simulink model "CubeRF"  (R2020b)
settings: Solver=FixedStepAuto  StartTime=0.0  StopTime=inf  FixedStep=0.05  RelTol=1e-3
undefined symbols (not defined in the file): Pose, Twist
libraries: robotlib x3
settings Model: Creator=iris  LastModifiedBy=iris
settings OptimizationCC: EnhancedBackFolding=on  PassReuseOutputArgsAs=Individual arguments  ZeroExternalMemoryAtStartup=off  ZeroInternalMemoryAtStartup=off  MaxStackSize=64  OptimizeBlockOrder=speed  DifferentSizesBufferReuse=on  OptimizationCustomize=off  EfficientTunableParamExpr=on
settings DebuggingCC: ParameterTunabilityLossMsg=error  SFMachineParentedDataDiag=error
settings HardwareCC: ProdBitPerPointer=32  ProdBitPerSizeT=32  ProdBitPerPtrDiffT=32  ProdLargestAtomicFloat=None  ProdIntDivRoundTo=Undefined  ProdEndianess=Unspecified  ProdWordSize=32  ProdHWDeviceType=Generic->Unspecified (assume 32-bit Generic)
settings SFSimCC: MATLABDynamicMemAlloc=off  SimTargetLang=C++
settings RTWCC: Description=Embedded Coder  SystemTargetFile=ert.tlc  HardwareBoard=Robot Operating System (ROS)  TLCOptions="-aInlineSetEventsForThisBaseRateFcn=TLC_FALSE -aSuppressMultiTaskScheduler=TLC_FALSE  -aRateBasedStepFcn=0"  TemplateMakefile=ert_default_tmf  Toolchain=Catkin  TargetLang=C++
settings CodeAppCC: ForceParamTrailComments=on  IgnoreCustomStorageClasses=off  OperatorAnnotations=on  SimulinkDataObjDesc=on  SFDataObjDesc=on  InsertBlockDesc=on
settings ERTTargetCC: SupportVariableSizeSignals=on

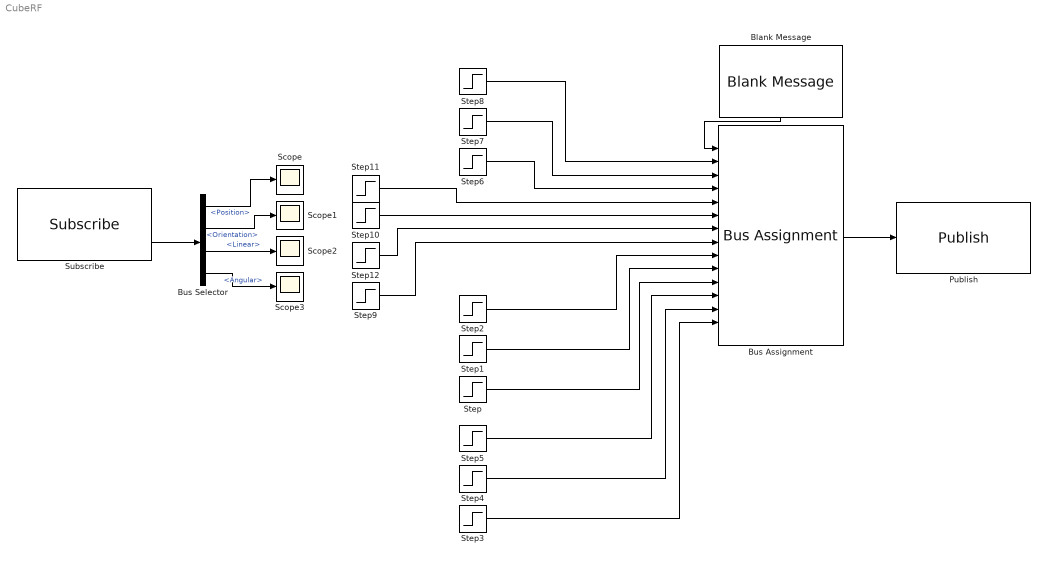
== system CubeRF ==
  Blank Message : robotlib/Blank Message  messageClass=Message  entityType=nav_msgs/Odometry  messageType=nav_msgs/Odometry  SampleTime=inf  legacyBusStruct=off
  Bus Assignment : BusAssignment  AssignedSignals=Pose.Pose.Position.X,Pose.Pose.Position.Y,Pose.Pose.Position.Z,Pose.Pose.Orientation.X,Pose.Pose.Orientation.Y,Pose.Pose.Orientation.Z,Pose.Pose.Orientation.W,Twist.Twist.Linear.X,Twist.Twist.Linear.Y,Twist.Twist.Linear.Z,Twist.Twist.Angular.X,Twist.Twist.Angular.Y,Twist.Twist.Angular.Z
  Bus Selector : BusSelector  OutputSignals=Pose.Pose.Position,Pose.Pose.Orientation,Twist.Twist.Linear,Twist.Twist.Angular
  Publish : robotlib/Publish  topicSource=Specify your own  topic=/CubeCommand  messageType=nav_msgs/Odometry  legacyBusStruct=off  messageQueueLength=1
  Scope{,1..3} (4 alike) : Scope
  Step{,1..8,10..11} (11 alike) : Step  After=0  SampleTime=0
  Step12 : Step  After=0.7  SampleTime=0
  Step9 : Step  After=0.7  SampleTime=0
  Subscribe : robotlib/Subscribe  topicSource=Specify your own  topic=/odom  messageType=nav_msgs/Odometry  SampleTime=-1  legacyBusStruct=off  messageQueueLength=1
  wires:
  Bus Assignment/1 -> Publish/1
  Blank Message/1 -> Bus Assignment/1
  Subscribe/2 -> Bus Selector/1
  Bus Selector/1 -> Scope/1  "<Position>"
  Bus Selector/2 -> Scope1/1  "<Orientation>"
  Bus Selector/3 -> Scope2/1  "<Linear>"
  Bus Selector/4 -> Scope3/1  "<Angular>"
  Step2/1 -> Bus Assignment/9
  Step1/1 -> Bus Assignment/10
  Step/1 -> Bus Assignment/11
  Step5/1 -> Bus Assignment/12
  Step4/1 -> Bus Assignment/13
  Step3/1 -> Bus Assignment/14
  Step8/1 -> Bus Assignment/2
  Step7/1 -> Bus Assignment/3
  Step6/1 -> Bus Assignment/4
  Step11/1 -> Bus Assignment/5
  Step10/1 -> Bus Assignment/6
  Step9/1 -> Bus Assignment/8
  Step12/1 -> Bus Assignment/7
